simulink model "nanogrid_model"  (R2022a)
settings: Solver=VariableStepAuto  StartTime=0.0  StopTime=86000  RelTol=1e-3
undefined symbols (not defined in the file): Ion, Lithium, sigbuilder_block
libraries: spsCurrentMeasurementLib x18, spsControlledCurrentSourceLib x16, spsVoltageMeasurementLib x12, spsParallelRLCBranchLib x2, spsVariableResistorLib x2, spsBatteryLib x2, spsPVArrayLib x2, spsControlledVoltageSourceLib x1, spsSeriesRLCBranchLib x1, spspowerguiLib x1
(part 1 of 2)
settings Model: SnapshotBufferSize=10000  PacingRate=10  Creator=mhenk  LastModifiedBy=mhenk

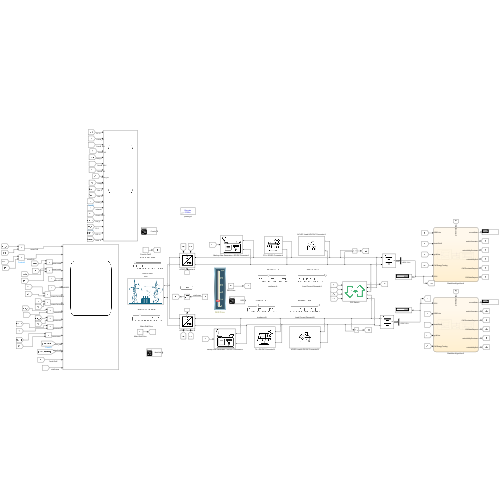
[thumbnail: Simulink's stored preview of the top-level diagram]
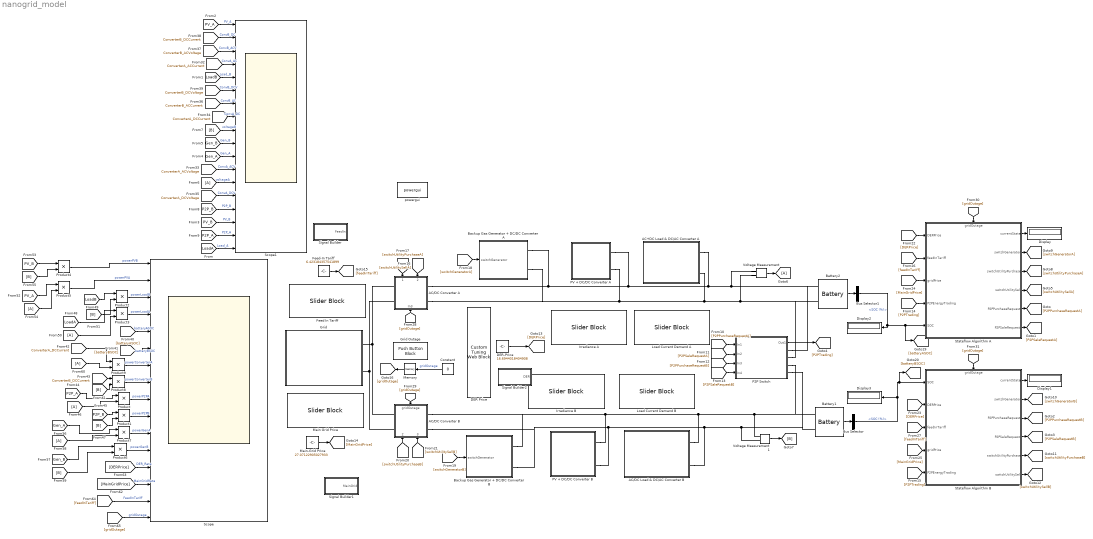
== system nanogrid_model ==
  AC+DC Load & DC/AC Converter A : Subsystem
      mask Display: image('C:\Users\mhenk\Desktop\Data Sync\Documents\education\HSU-UniBwH\Master Thesis\MatLab\own stuff\matlab icons\house load icon.png'); % Use "Edit Image" on toolstrip to change.
  AC/DC Converter A : Subsystem
      settings: PortSchema="{\"entries\":[{\"content\":{\"sides\":[{\"content\":{\"connectorIds\":[\"LConn1\",\"LConn2\"]},\"type\":\"ConnectorPlacement.EquallySpacedRectSide\",\"uuid\":\"d108abb1-5086-446c-b15f-f019b5d6e838\"},{\"content\":{\"connectorIds\":[\"RConn1\",\"RConn2\"],\"side\":\"RIGHT\"},\"type\":\"ConnectorPlacement.EquallySpacedRectSide\",\"uuid\":\"21957a4b-95ce-4ceb-ba72-e824460ef8fd\"},{\"content\":{\"connectorIds\":[\"In1\",\"In2\"],\"side\":\"TOP\"},\"type\":\"ConnectorPlacement.EquallySpacedRectSide\",\"uuid\":\"459c1e26-38cf-4009-a7ae-852720303eb2\"},{\"content\":{\"connectorIds\":[\"In3\"],\"side\":\"BOTTOM\"},\"type\":\"ConnectorPlacement.EquallySpacedRectSide\",\"uuid\":\"e1e3ddba-a993-4c48-8674-2bf20986e444\"}]},\"type\":\"ConnectorPlacement.EquallySpacedConnector\",\"uuid\":\"dcdecdb1-f7ff-4942-94d1-dadc92311a87\"}],\"packageUris\":[\"http://schema.mathworks.com/mf0/Connector/R2020b\"],\"version\":\"1.0\"}"
      mask Display: image('C:\Users\mhenk\Desktop\Data Sync\Documents\education\HSU-UniBwH\Master Thesis\MatLab\own stuff\matlab icons\ac dc converter.png'); % Use "Edit Image" on toolstrip to change.
  AC/DC Converter B : Subsystem
      settings: PortSchema="{\"entries\":[{\"content\":{\"sides\":[{\"content\":{\"connectorIds\":[\"LConn1\",\"LConn2\"]},\"type\":\"ConnectorPlacement.EquallySpacedRectSide\",\"uuid\":\"d108abb1-5086-446c-b15f-f019b5d6e838\"},{\"content\":{\"connectorIds\":[\"RConn1\",\"RConn2\"],\"side\":\"RIGHT\"},\"type\":\"ConnectorPlacement.EquallySpacedRectSide\",\"uuid\":\"21957a4b-95ce-4ceb-ba72-e824460ef8fd\"},{\"content\":{\"connectorIds\":[\"In1\"],\"side\":\"TOP\"},\"type\":\"ConnectorPlacement.EquallySpacedRectSide\",\"uuid\":\"459c1e26-38cf-4009-a7ae-852720303eb2\"},{\"content\":{\"connectorIds\":[\"In2\",\"In3\"],\"side\":\"BOTTOM\"},\"type\":\"ConnectorPlacement.EquallySpacedRectSide\",\"uuid\":\"e1e3ddba-a993-4c48-8674-2bf20986e444\"}]},\"type\":\"ConnectorPlacement.EquallySpacedConnector\",\"uuid\":\"dcdecdb1-f7ff-4942-94d1-dadc92311a87\"}],\"packageUris\":[\"http://schema.mathworks.com/mf0/Connector/R2020b\"],\"version\":\"1.0\"}"
      mask Display: image('C:\Users\mhenk\Desktop\Data Sync\Documents\education\HSU-UniBwH\Master Thesis\MatLab\own stuff\matlab icons\ac dc converter.png'); % Use "Edit Image" on toolstrip to change.
  AC/DC Load & DC/AC Converter B : Subsystem
      mask Display: image('C:\Users\mhenk\Desktop\Data Sync\Documents\education\HSU-UniBwH\Master Thesis\MatLab\own stuff\matlab icons\house load icon.png'); % Use "Edit Image" on toolstrip to change.
  Backup Gas Generator + DC/DC Converter A : Subsystem
      mask Display: image('C:\Users\mhenk\Desktop\Data Sync\Documents\education\HSU-UniBwH\Master Thesis\MatLab\own stuff\matlab icons\gas generator.jpg'); % Use "Edit Image" on toolstrip to change.
  Backup Gas Generator + DC/DC Converter B : Subsystem
      mask Display: image('C:\Users\mhenk\Desktop\Data Sync\Documents\education\HSU-UniBwH\Master Thesis\MatLab\own stuff\matlab icons\gas generator.jpg'); % Use "Edit Image" on toolstrip to change.
  Battery1 : spsBatteryLib/Battery  BatType=Lithium-Ion  ShowTempParam=off  ThermalPreset="12.8V  40Ah  (LiFeMgPO4)"  ShowAgeParam=off  NomV=24  NomQ=500  SOC=1.1  Batt_Tr=30  PresetModel=on  MaxQ=500  MinV=18  FullV=27.9357  Dis_rate=217.3913  R=0.00048  Normal_OP=452.1739  expZone="[25.9293      24.5652]"  current=[6.5 13 32.5]  Units=Time  Tci=20  NomT=20  T2=0  MaxQ2=36  FullV2=13  Normal_OP2=11.7  expZone2="[12.67            4]"  Rca=0.6411  ti=4880  Dp=0  Neq0=0  Tsim=1e6  Ta1=25  Qeol=5.4*0.9  Reol=0.013333*1.2  Char_age=[2.3478, 3]  Dis_age=[2.3478, 10]  N1=1500  N2=10500  N3=1000  N4=1400  Ta2=45  N5=950
  Battery2 : spsBatteryLib/Battery  BatType=Lithium-Ion  ShowTempParam=off  ThermalPreset="12.8V  40Ah  (LiFeMgPO4)"  ShowAgeParam=off  NomV=24  NomQ=500  SOC=99  Batt_Tr=30  PresetModel=on  MaxQ=500  MinV=18  FullV=27.9357  Dis_rate=217.3913  R=0.00048  Normal_OP=452.1739  expZone="[25.9293      24.5652]"  current=[6.5 13 32.5]  Units=Time  Tci=20  NomT=20  T2=0  MaxQ2=36  FullV2=13  Normal_OP2=11.7  expZone2="[12.67            4]"  Rca=0.6411  ti=4880  Dp=0  Neq0=0  Tsim=1e6  Ta1=25  Qeol=5.4*0.9  Reol=0.013333*1.2  Char_age=[2.3478, 3]  Dis_age=[2.3478, 10]  N1=1500  N2=10500  N3=1000  N4=1400  Ta2=45  N5=950
  Bus Selector : BusSelector  OutputSignals=SOC (%)
  Bus Selector1 : BusSelector  OutputSignals=SOC (%)
  Constant : Constant  Value=0
  DER Price : CustomTuningWebBlock  LabelPosition=Hide  ShowInitialText=on  Configuration="{\"type\":\"LinearGauge\",\"settings\":{\"BindingType\":\"param\",\"aspectRatio\":3.7777777777777777,\"backgroundColor\":[0,0,0,\"1\"],\"backgroundOffset\":0,\"backgroundOpacity\":1,\"fixedAspectRatio\":\"on\",\"foregroundColor\":[252,252,196],\"orientation\":\"vertical\",\"showBackgroundColor\":false,\"value\":0},\"components\":[{\"name\":\"LinearScaleComponent\",\"settings\":{\"bounds\":{\"max\":100,\"min\":1,\"tickInterval\":\"auto\"},\"internalTickHeightScaleFactor\":0.5,\"labelColor\":[255,255,200],\"labelFont\":{\"font\":\"Arial\",\"fontSize\":12},\"labelTransparency\":1,\"needleImage\":{\"size\":[596,842],\"src\":\"data:image/svg+xml;base64,PD94bWwgdmVyc2lvbj0iMS4wIiBlbmNvZGluZz0idXRmLTgiPz4NCjwhLS0gR2VuZXJhdG9yOiBBZG9iZSBJbGx1c3RyYXRvciAyNS4wLjAsIFNWRyBFeHBvcnQgUGx1Zy1JbiAuIFNWRyBWZXJzaW9uOiA2LjAwIEJ1aWxkIDApICAtLT4NCjxzdmcgdmVyc2lvbj0iMS4xIg0KCSBpZD0ic3ZnOCIgeG1sbnM6Y2M9Imh0dHA6Ly9jcmVhdGl2ZWNvbW1vbnMub3JnL25zIyIgeG1sbnM6ZGM9Imh0dHA6Ly9wdXJsLm9yZy9kYy9lbGVtZW50cy8xLjEvIiB4bWxuczppbmtzY2FwZT0iaHR0cDovL3d3dy5pbmtzY2FwZS5vcmcvbmFtZXNw ...(+2420 chars)\",\"srcOrientation\":\"horizontal\"},\"needleOffset\":[0.0642123287671233,-0.8044596912521441],\"needleSize\":{\"height\":0.07668067226890757,\"width\":0.4337797619047619},\"position\":[0.03607382550335571,0.2824519230769231,0.6089743589743589,0.9195679530201343],\"referencePoint\":\"auto\",\"scaleColors\":[],\"scaleColorsSize\":0.2,\"scaleDirection\":\"BT\",\"showLabels\":1,\"showMinorTicks\":0,\"showSpanLine\":1,\"showTicks\":1,\"tickColor\":[252,252,197],\"tickTransparency\":1,\"valueBarColor\":[0,114,189],\"valueBarOffset\":-0.27,\"valueBarSize\":0.1,\"valueBarTransparency\":1}},{\"name\":\"BackgroundImageComponent\",\"settings\":{\"image\":{\"size\":[380,101],\"src\":\"data:image/svg+xml;base64,PHN2ZyB4bWxucz0iaHR0cDovL3d3dy53My5vcmcvMjAwMC9zdmciIHhtbG5zOnhsaW5rPSJodHRwOi8vd3d3LnczLm9yZy8xOTk5L3hsaW5rIiB2aWV3Qm94PSIwIDAgMzgwIDEwMSI+PGRlZnM+PHN0eWxlPi5jbHMtMXtmaWxsOiMwMDJiNDI7fS5jbHMtMntmaWxsOiM0MjcwODI7fS5jbHMtM3tmaWxsOnVybCgjcmFkaWFsLWdyYWRpZW50KTt9LmNscy00e2ZpbGw6I2M4YzhjODtzdHJva2U6IzAwMDt9PC9zdHlsZT48cmFkaWFsR3JhZGllbnQgaWQ9InJhZGlhbC1ncmFkaWVudCIgY3g9IjE5MCIgY3k9IjUwLjUiIHI9IjI2OS4yMSIgZ3JhZGllbnRVbml0cz0idXNlclNwYWNlT25Vc2UiPjxzdG9wIG9mZnNldD0iMC4wMSIgc3RvcC1jb2xvcj0iIzNlNGY1OCIvPjxzdG9wIG9mZnNldD0iMC4wNiIgc3RvcC1jb2xvcj0iIzQ0NTc2MSIvPjxzdG9wIG9mZnNldD0iMC4xNSIgc3RvcC1jb2xvcj0iIzU1NmE3NiIvPjxzdG9wIG9mZnNldD0iMC4yNSIgc3RvcC1jb2xvcj0iIzZkODg5NSIvPjxzdG9wIG9mZnNldD0iMC4zOCIgc3RvcC1jb2xvcj0iIzhmYjJjMyIvPjxzdG9wIG9mZnNldD0iMC41MiIgc3RvcC1jb2xvcj0iI2I2ZTRmYSIvPjxzdG9wIG9mZnNldD0iMSIgc3RvcC1jb2xvcj0iIzE1NDY1NyIvPjwvcmFkaWFsR3JhZGllbnQ+PC9kZWZzPjxnIGlkPSJmcmFtZSI+PGcgaWQ9IkxheWVyXzIiIGRhdGEtbmFtZT0iTGF5ZXIgMiI+PGcgaWQ9IkxheWVyXzEtMiIgZGF0YS1uYW1lPSJMYXllciAxLTIiPjxyZWN0IGlkPSJyZWN0MTAzNiIgY2xhc3M9ImNscy0xIiB4PSIxMSIgeT0iMTEiIHdpZHRoPSIzNTgiIGhlaWdodD0iNzkiLz48cGF0aCBpZD0icGF0aDEwMzgiIGNsYXNzPSJjbHMtMiIgZD0iTTgsOFY5M0gzNzJWOFpNMzY5LDkwSDExVjExSDM2OVoiLz48cGF0aCBpZD0icGF0aDEwNDAiIGNsYXNzPSJjbHMtMyIgZD0iTTAsMFYxMDFIMzgwVjBaTTM3Miw5M0g4VjhIMzcyWiIvPjwvZz48L2c+PC9nPjxnIGlkPSJ0cmFjayI+PHBhdGggaWQ9InJlY3QxNjExIiBjbGFzcz0iY2xzLTQiIGQ9Ik0zMy4zNywyNi41OUgzNDYuNjNjNCwwLDcuMjUsMi42LDcuMjUsNS44MWgwYzAsMy4yMS0zLjI1LDUuODItNy4yNSw1LjgySDMzLjM3Yy00LDAtNy4yNS0yLjYxLTcuMjUtNS44MmgwQzI2LjEyLDI5LjE5LDI5LjM3LDI2LjU5LDMzLjM3LDI2LjU5WiIvPjwvZz48L3N2Zz4=\",\"srcOrientation\":\"horizontal\"},\"position\":[0,0,1,1],\"scaleMode\":\"0\"}},{\"name\":\"ForegroundImageComponent\",\"settings\":{\"image\":{\"size\":[0,0],\"src\":\"default\",\"srcOrientation\":[]},\"isForeground\":1,\"position\":[0,0,1,1],\"scaleMode\":\"0\"}}]}"
  DER-Price : Constant  Value=16.6944018404908
  Display{,1..3} (4 alike) : Display
  Feed In Tariff : SliderBlock  ScaleMin=1
  Feed-In Tariff : Constant  Value=6.423184357541899
  From{6,46,50,54,58,60} (6 alike) : From
  Goto6 : Goto
  Grid : Subsystem
      mask Display: image('C:\Users\mhenk\Desktop\Data Sync\Documents\education\HSU-UniBwH\Master Thesis\MatLab\own stuff\matlab icons\power grid transformer substation.jpg'); % Use "Edit Image" on toolstrip to change.
  Grid Outage : PushButtonBlock  ButtonType=Latch  OffValue=0.000000
  Irradiance A : SliderBlock  ScaleMax=1000
  Irradiance B : SliderBlock  ScaleMax=1000
  Load Current Demand A : SliderBlock
  Load Current Demand B : SliderBlock
  Main Grid Price : SliderBlock  ScaleMin=1
  Main-Grid Price : Constant  Value=27.07122905027933
  Memory : Memory
  P2P Switch : Subsystem
      mask Display: image('C:\Users\mhenk\Desktop\Data Sync\Documents\education\HSU-UniBwH\Master Thesis\MatLab\own stuff\matlab icons\p2p.png'); % Use "Edit Image" on toolstrip to change.
  PV + DC/DC Converter A : Subsystem
      mask Display: image('C:\Users\mhenk\Desktop\Data Sync\Documents\education\HSU-UniBwH\Master Thesis\MatLab\own stuff\matlab icons\pv icon.png'); % Use "Edit Image" on toolstrip to change.
  PV + DC/DC Converter B : Subsystem
      mask Display: image('C:\Users\mhenk\Desktop\Data Sync\Documents\education\HSU-UniBwH\Master Thesis\MatLab\own stuff\matlab icons\pv icon.png'); % Use "Edit Image" on toolstrip to change.
  Product{,1..9} (10 alike) : Product
  Scope : Scope  NumInputPorts=16
  Scope1 : Scope  NumInputPorts=18
  Signal Builder : Subsystem  Tag=STV Subsys  LoadFcn=sigbuilder_block('load');  StartFcn=sigbuilder_block('start');  StopFcn=sigbuilder_block('stop');  ClipboardFcn=sigbuilder_block('clipboard');  mask(Sigbuilder block){tuvar=[0:10]}
      mask help: Simulink:masks:SigbuilderBlock_MD
      mask init:
      | if ~strcmp(get_param(bdroot(gcbh),'SimulationStatus'),'stopped') tuvar = sigbuilder_block('maskInit'); end
      settings: CopyFcn=sigbuilder_block('copy');  DeleteFcn=sigbuilder_block('delete');  ModelCloseFcn=sigbuilder_block('modelClose');  PreSaveFcn=sigbuilder_block('preSave');  PauseFcn=sigbuilder_block('pause');  ContinueFcn=sigbuilder_block('continue');  NameChangeFcn=sigbuilder_block('namechange');  OpenFcn=sigbuilder_block('open',[426.6 153 550.8 400.2 ]);  CloseFcn=sigbuilder_block('close');
      mask Display: plot(0, 0, 100, 100,[2, 2, 32, 32, 2], [68, 8, 8, 68, 68],[32, 2], [38, 38], [32, 19, 2],[53, 60, 44], [32, 17, 17, 2],[16, 16, 31, 31]);txt = getActiveGroup(gcbh);text(2, 100, txt,'verticalAlignment', 'top');
  Signal Builder1 : Subsystem  Tag=STV Subsys  LoadFcn=sigbuilder_block('load');  StartFcn=sigbuilder_block('start');  StopFcn=sigbuilder_block('stop');  ClipboardFcn=sigbuilder_block('clipboard');  mask(Sigbuilder block){tuvar=[0:10]}
      mask help: Simulink:masks:SigbuilderBlock_MD
      mask init:
      | if ~strcmp(get_param(bdroot(gcbh),'SimulationStatus'),'stopped') tuvar = sigbuilder_block('maskInit'); end
      settings: CopyFcn=sigbuilder_block('copy');  DeleteFcn=sigbuilder_block('delete');  ModelCloseFcn=sigbuilder_block('modelClose');  PreSaveFcn=sigbuilder_block('preSave');  PauseFcn=sigbuilder_block('pause');  ContinueFcn=sigbuilder_block('continue');  NameChangeFcn=sigbuilder_block('namechange');  OpenFcn=sigbuilder_block('open',[426.6 153 550.8 400.2 ]);  CloseFcn=sigbuilder_block('close');
      mask Display: plot(0, 0, 100, 100,[2, 2, 32, 32, 2], [68, 8, 8, 68, 68],[32, 2], [38, 38], [32, 19, 2],[53, 60, 44], [32, 17, 17, 2],[16, 16, 31, 31]);txt = getActiveGroup(gcbh);text(2, 100, txt,'verticalAlignment', 'top');
  Signal Builder2 : Subsystem  Tag=STV Subsys  LoadFcn=sigbuilder_block('load');  StartFcn=sigbuilder_block('start');  StopFcn=sigbuilder_block('stop');  ClipboardFcn=sigbuilder_block('clipboard');  mask(Sigbuilder block){tuvar=[0:10]}
      mask help: Simulink:masks:SigbuilderBlock_MD
      mask init:
      | if ~strcmp(get_param(bdroot(gcbh),'SimulationStatus'),'stopped') tuvar = sigbuilder_block('maskInit'); end
      settings: CopyFcn=sigbuilder_block('copy');  DeleteFcn=sigbuilder_block('delete');  ModelCloseFcn=sigbuilder_block('modelClose');  PreSaveFcn=sigbuilder_block('preSave');  PauseFcn=sigbuilder_block('pause');  ContinueFcn=sigbuilder_block('continue');  NameChangeFcn=sigbuilder_block('namechange');  OpenFcn=sigbuilder_block('open',[426.6 153 550.8 400.2 ]);  CloseFcn=sigbuilder_block('close');
      mask Display: plot(0, 0, 100, 100,[2, 2, 32, 32, 2], [68, 8, 8, 68, 68],[32, 2], [38, 38], [32, 19, 2],[53, 60, 44], [32, 17, 17, 2],[16, 16, 31, 31]);txt = getActiveGroup(gcbh);text(2, 100, txt,'verticalAlignment', 'top');
  Stateflow Algorithm A : Stateflow chart  TreatAsAtomicUnit=on
      settings: PortSchema="{\"entries\":[{\"content\":{\"sides\":[{\"content\":{\"connectorIds\":[\"In3\",\"In4\",\"In5\",\"In6\",\"In2\"]},\"type\":\"ConnectorPlacement.EquallySpacedRectSide\",\"uuid\":\"fa40be95-7d12-4090-b6c9-44da1494b39c\"},{\"content\":{\"connectorIds\":[\"Out1\",\"Out2\",\"Out3\",\"Out4\",\"Out5\",\"Out6\"],\"side\":\"RIGHT\"},\"type\":\"ConnectorPlacement.EquallySpacedRectSide\",\"uuid\":\"baf17cd9-68a7-482b-a40a-ea138c452546\"},{\"content\":{\"connectorIds\":[\"In1\"],\"side\":\"TOP\"},\"type\":\"ConnectorPlacement.EquallySpacedRectSide\",\"uuid\":\"87fda98d-0e45-402d-8086-d8aba4cb4e5b\"}]},\"type\":\"ConnectorPlacement.EquallySpacedConnector\",\"uuid\":\"afd8760f-ef20-4593-b581-61316121c6e0\"}],\"packageUris\":[\"http://schema.mathworks.com/mf0/Connector/R2020b\"],\"version\":\"1.0\"}"
  Stateflow Algorithm B : Stateflow chart  TreatAsAtomicUnit=on
      settings: PortSchema="{\"entries\":[{\"content\":{\"sides\":[{\"content\":{\"connectorIds\":[\"In2\",\"In3\",\"In4\",\"In5\",\"In6\"]},\"type\":\"ConnectorPlacement.EquallySpacedRectSide\",\"uuid\":\"222fe6c9-2492-4286-b2fe-ee0502c7d1b1\"},{\"content\":{\"connectorIds\":[\"Out1\",\"Out2\",\"Out3\",\"Out4\",\"Out5\",\"Out6\"],\"side\":\"RIGHT\"},\"type\":\"ConnectorPlacement.EquallySpacedRectSide\",\"uuid\":\"fe6cecda-2536-4b6e-a5a3-681bec7accbb\"},{\"content\":{\"connectorIds\":[\"In1\"],\"side\":\"TOP\"},\"type\":\"ConnectorPlacement.EquallySpacedRectSide\",\"uuid\":\"dd9ad14a-77c7-4598-a0b7-e283792e3e97\"}]},\"type\":\"ConnectorPlacement.EquallySpacedConnector\",\"uuid\":\"4279e8cf-6645-4663-97ae-cc11306bf231\"}],\"packageUris\":[\"http://schema.mathworks.com/mf0/Connector/R2020b\"],\"version\":\"1.0\"}"
  Voltage Measurement : spsVoltageMeasurementLib/Voltage Measurement  PhasorSimulation=off  OutputType=Complex  PSBequivalent=0
  Voltage Measurement1 : spsVoltageMeasurementLib/Voltage Measurement  PhasorSimulation=off  OutputType=Complex  PSBequivalent=0
  powergui : spspowerguiLib/powergui  Priority=1  SimulationMode=Discrete  SampleTime=0.009  frequency=50  Iterations=50  frequencyindice=0  Pbase=100e6  ErrMax=1e-4  UnitsV=kV  UnitsW=MW  buscounter=0  FunctionMessages=off  echomessages=off  EnableUseOfTLC=off  CurrentSourceSwitches=off  DisableSnubberDevices=off  DisableRonSwitches=off  DisableVfSwitches=off  DisplayEquations=off  AutomaticDiscreteSolvers=off  SolverType=Tustin/Backward Euler (TBE)  Interpol=off  ExternalGateDelay=off  methode=off  Ts=100  x0status=blocks  SPID=on  SwTol=0  HookPort=off  NonlinearTolerance=1e-4  nMaxIteration=100  ContinueOnMaxIteration=off  RestoreLinks=warning  ResistiveCurrentMeasurement=off  Frange=[0:2:500]  Ylog=off  Xlog=on  ShowGrid=off  save=off  variable=ZData  structure=0  ZoomFFT=off  StartTime=0.0  cycles=1  DisplayStyle=1  fundamental=60  FreqAxis=off  MaxFrequency=1000  frequencyindicesteady=1  RmsSteady=1  display=off
  wires:
  Battery1/1 -> Bus Selector/1
  Battery2/1 -> Bus Selector1/1
  Bus Selector/1 -> [batteryBSOC], Stateflow Algorithm B/2(SOC), Display3/1  "<SOC (%)>"
  Bus Selector1/1 -> [batteryASOC], Stateflow Algorithm A/2(SOC), Display2/1  "<SOC (%)>"
  Voltage Measurement/1 -> Goto6/1
  Stateflow Algorithm A/1(currentState) -> Display/1
  Stateflow Algorithm B/1(currentState) -> Display1/1
  Voltage Measurement1/1 -> [B]
  Stateflow Algorithm A/5(P2PPurchaseRequest) -> [P2PPurchaseRequestA]
  [P2PPurchaseRequestA] -> P2P Switch/1(In1)
  [P2PSaleRequestA] -> P2P Switch/2(In2)
  Stateflow Algorithm A/6(P2PSaleRequest) -> [P2PSaleRequestA]
  Stateflow Algorithm B/3(P2PPurchaseRequest) -> [P2PPurchaseRequestB]
  [P2PPurchaseRequestB] -> P2P Switch/3(In3)
  Stateflow Algorithm B/4(P2PSaleRequest) -> [P2PSaleRequestB]
  [P2PSaleRequestB] -> P2P Switch/4(In4)
  [P2PTrading] -> Stateflow Algorithm A/6(P2PEnergyTrading)
  [P2PTrading] -> Stateflow Algorithm B/6(P2PEnergyTrading)
  P2P Switch/1(Out1) -> [P2PTrading]
  Stateflow Algorithm A/4(switchUtilitySell) -> [switchUtilitySellA]
  [switchUtilitySellA] -> AC/DC Converter A/2(switchGridSell)
  [switchUtilityPurchaseA] -> AC/DC Converter A/1(switchGridPurchase)
  Stateflow Algorithm A/3(switchUtilityPurchase) -> [switchUtilityPurchaseA]
  Stateflow Algorithm A/2(switchGenerator) -> [switchGeneratorA]
  [switchGeneratorA] -> Backup Gas Generator + DC/DC Converter A/1(switchGenerator)
  [switchGeneratorB] -> Backup Gas Generator + DC/DC Converter B/1(switchGenerator)
  Stateflow Algorithm B/2(switchGenerator) -> [switchGeneratorB]
  Stateflow Algorithm B/5(switchUtilityPurchase) -> [switchUtilityPurchaseB]
  [switchUtilityPurchaseB] -> AC/DC Converter B/2(switchGridPurchase)
  [switchUtilitySellB] -> AC/DC Converter B/3(switchGridSell)
  Stateflow Algorithm B/6(switchUtilitySell) -> [switchUtilitySellB]
  [DERPrice] -> Stateflow Algorithm A/3(DERPrice)
  [DERPrice] -> Stateflow Algorithm B/3(DERPrice)
  [MainGridPrice] -> Stateflow Algorithm A/5(gridPrice)
  [MainGridPrice] -> Stateflow Algorithm B/5(gridPrice)
  [feedInTariff] -> Stateflow Algorithm A/4(feedInTariff)
  [feedInTariff] -> Stateflow Algorithm B/4(feedInTariff)
  Memory/1 -> [gridOutage]
  [gridOutage] -> AC/DC Converter A/3(In3)
  [gridOutage] -> AC/DC Converter B/1(gridOutage)
  [PV_A] -> Scope1/1  "PV_A"
  [LoadA] -> Scope1/18  "Load_A"
  [LoadB] -> Scope1/5  "Load_B"
  [gridOutage] -> Stateflow Algorithm A/1(gridOutage)
  [gridOutage] -> Stateflow Algorithm B/1(gridOutage)
  [B] -> Product1/2
  [P2P_B] -> Product1/1
  Product1/1 -> Scope/10  "powerP2PB"
  From50/1 -> Product3/2
  [LoadA] -> Product3/1
  [LoadB] -> Product2/1
  [B] -> Product2/2
  [B] -> Product4/2
  [PV_B] -> Product4/1
  From58/1 -> Product7/2
  [Gen_A] -> Product7/1
  [B] -> Product6/2
  [Gen_B] -> Product6/1
  Product7/1 -> Scope/11  "powerGenA"
  Product6/1 -> Scope/12  "powerGenB"
  Product2/1 -> Scope/3  "powerLoadB"
  Product3/1 -> Scope/4  "powerLoadA"
  Product4/1 -> Scope/1  "powerPVB"
  Constant/1 -> Memory/1  "gridOutage"
  [B] -> Product8/2
  [ConverterA_DCCurrent] -> Product9/1
  From60/1 -> Product9/2
  [ConverterB_DCCurrent] -> Product8/1
  Product9/1 -> Scope/7  "powerConverterA"
  Product8/1 -> Scope/8  "powerConverterB"
  [PV_B] -> Scope1/16  "PV_B"
  [Gen_B] -> Scope1/10  "Gen_B"
  [Gen_A] -> Scope1/11  "Gen_A"
  [P2P_B] -> Scope1/15  "P2P_B"
  [P2P_A] -> Scope1/17  "P2P_A"
  From6/1 -> Scope1/13  "voltageA"
  [ConverterA_ACVoltage] -> Scope1/12  "ConvA_ACV"
  [ConverterA_DCCurrent] -> Scope1/8  "ConvA_DC"
  [B] -> Scope1/9  "voltageB"
  [batteryASOC] -> Scope/5  "batteryASOC"
  [ConverterA_DCVoltage] -> Scope1/14  "ConvA_DCV"
  [ConverterA_ACCurrent] -> Scope1/4  "ConvA_AC"
  [ConverterB_ACCurrent] -> Scope1/7  "ConvB_AC"
  [ConverterB_DCCurrent] -> Scope1/2  "ConvB_DC"
  [ConverterB_DCVoltage] -> Scope1/6  "ConvB_DCV"
  [ConverterB_ACVoltage] -> Scope1/3  "ConvB_ACV"
  [P2P_A] -> Product/1
  From46/1 -> Product/2
  Product/1 -> Scope/9  "powerP2PA"
  [PV_A] -> Product5/1
  From54/1 -> Product5/2
  Product5/1 -> Scope/2  "powerPVA"
  [batteryBSOC] -> Scope/6  "batteryBSOC"
  [DERPrice] -> Scope/13  "DER_Rate"
  [MainGridPrice] -> Scope/14  "MainGridRate"
  [feedInTariff] -> Scope/15  "FeedInTariff"
  [gridOutage] -> Scope/16  "gridOutage"
  Feed-In Tariff/1 -> [feedInTariff]
  Main-Grid Price/1 -> [MainGridPrice]
  DER-Price/1 -> [DERPrice]
  connections:
  AC/DC Converter A/RConn1 -- Backup Gas Generator + DC/DC Converter A/RConn1 -- PV + DC/DC Converter A/RConn1 -- AC+DC Load & DC/AC Converter A/LConn1 -- P2P Switch/RConn1 -- Battery2/LConn1 -- Voltage Measurement/LConn1
  AC/DC Converter B/LConn2 -- AC/DC Converter A/LConn2 -- Grid/LConn2
  AC/DC Converter B/LConn1 -- AC/DC Converter A/LConn1 -- Grid/LConn1
  Voltage Measurement1/LConn1 -- Battery1/LConn1 -- P2P Switch/RConn3 -- Backup Gas Generator + DC/DC Converter B/RConn1 -- AC/DC Converter B/RConn1 -- PV + DC/DC Converter B/RConn1 -- AC/DC Load & DC/AC Converter B/RConn1
  Voltage Measurement/LConn2 -- P2P Switch/RConn2 -- Battery2/LConn2 -- AC/DC Converter A/RConn2 -- Backup Gas Generator + DC/DC Converter A/RConn2 -- PV + DC/DC Converter A/RConn2 -- AC+DC Load & DC/AC Converter A/LConn2
  AC/DC Load & DC/AC Converter B/RConn2 -- Battery1/LConn2 -- P2P Switch/RConn4 -- Voltage Measurement1/LConn2 -- Backup Gas Generator + DC/DC Converter B/RConn2 -- AC/DC Converter B/RConn2 -- PV + DC/DC Converter B/RConn2

== system nanogrid_model/AC+DC Load & DC//AC Converter A ==
  AC+DC Load & DC/AC Converter1 : Subsystem
  Current Measurement2 : spsCurrentMeasurementLib/Current Measurement  PhasorSimulation=off  OutputType=Complex  PSBequivalent=0
  Display : Display
  +1 : PMIOPort  Side=Left
  -1 : PMIOPort  Port=2  Side=Left
  tag scope: LoadA=global
  wires:
  Current Measurement2/1 -> Display/1, [LoadA]  "Load A current"
  connections:
  Current Measurement2/LConn1 -- AC+DC Load & DC/AC Converter1/LConn1
  Current Measurement2/RConn1 -- +1/RConn1
  AC+DC Load & DC/AC Converter1/LConn2 -- -1/RConn1

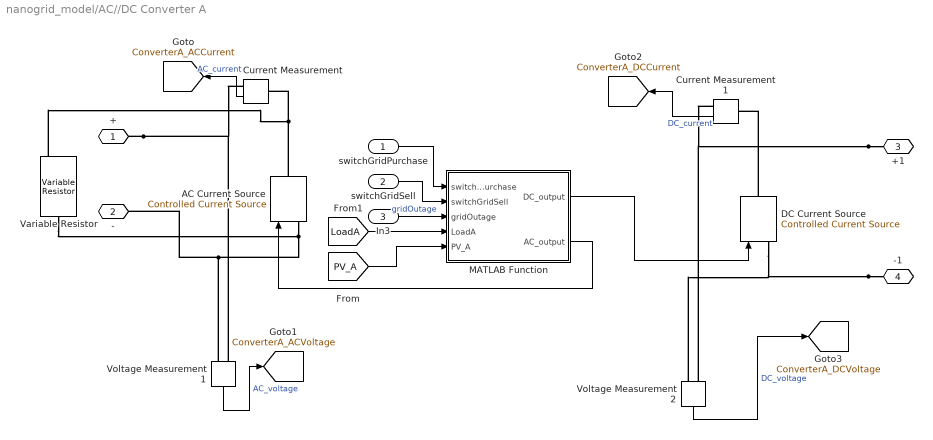
== system nanogrid_model/AC//DC Converter A ==
  switchGridPurchase : Inport
  switchGridSell : Inport  Port=2
  In3 : Inport  Port=3
  AC Current Source : spsControlledCurrentSourceLib/Controlled Current Source  Initialize=on  Source_Type=AC  Amplitude=0  Phase=0  Frequency=60  Measurements=None
  Current Measurement : spsCurrentMeasurementLib/Current Measurement  PhasorSimulation=off  OutputType=Complex  PSBequivalent=0
  Current Measurement1 : spsCurrentMeasurementLib/Current Measurement  PhasorSimulation=off  OutputType=Complex  PSBequivalent=0
  DC Current Source : spsControlledCurrentSourceLib/Controlled Current Source  Initialize=on  Source_Type=DC  Amplitude=0  Phase=0  Frequency=0  Measurements=None
  MATLAB Function : MATLAB Function  TreatAsAtomicUnit=on
  Variable Resistor : spsVariableResistorLib/Variable Resistor  Rabsmin=50e9
      settings: SourceProductBaseCode=PS
  Voltage Measurement1 : spsVoltageMeasurementLib/Voltage Measurement  PhasorSimulation=off  OutputType=Complex  PSBequivalent=0
  Voltage Measurement2 : spsVoltageMeasurementLib/Voltage Measurement  PhasorSimulation=off  OutputType=Complex  PSBequivalent=0
  + : PMIOPort  Side=Left
  - : PMIOPort  Port=2  Side=Left
  +1 : PMIOPort  Port=3  Side=Right
  -1 : PMIOPort  Port=4  Side=Right
  tag scope: ConverterA_ACCurrent=global, ConverterA_ACVoltage=global, ConverterA_DCCurrent=global, ConverterA_DCVoltage=global
  wires:
  MATLAB Function/1(DC_output) -> DC Current Source/1
  Current Measurement/1 -> [ConverterA_ACCurrent]  "AC_current"
  Voltage Measurement1/1 -> [ConverterA_ACVoltage]  "AC_voltage"
  Current Measurement1/1 -> [ConverterA_DCCurrent]  "DC_current"
  Voltage Measurement2/1 -> [ConverterA_DCVoltage]  "DC_voltage"
  MATLAB Function/2(AC_output) -> AC Current Source/1
  switchGridPurchase/1 -> MATLAB Function/1(switchGridPurchase)
  switchGridSell/1 -> MATLAB Function/2(switchGridSell)
  In3/1 -> MATLAB Function/3(gridOutage)  "gridOutage"
  [PV_A] -> MATLAB Function/5(PV_A)
  [LoadA] -> MATLAB Function/4(LoadA)
  connections:
  +/RConn1 -- Current Measurement/RConn1 -- Voltage Measurement1/LConn1
  AC Current Source/LConn1 -- Variable Resistor/RConn1 -- Voltage Measurement1/LConn2 -- -/RConn1
  AC Current Source/RConn1 -- Variable Resistor/LConn1 -- Current Measurement/LConn1
  -1/RConn1 -- Voltage Measurement2/LConn2 -- DC Current Source/LConn1
  +1/RConn1 -- Current Measurement1/RConn1 -- Voltage Measurement2/LConn1
  DC Current Source/RConn1 -- Current Measurement1/LConn1

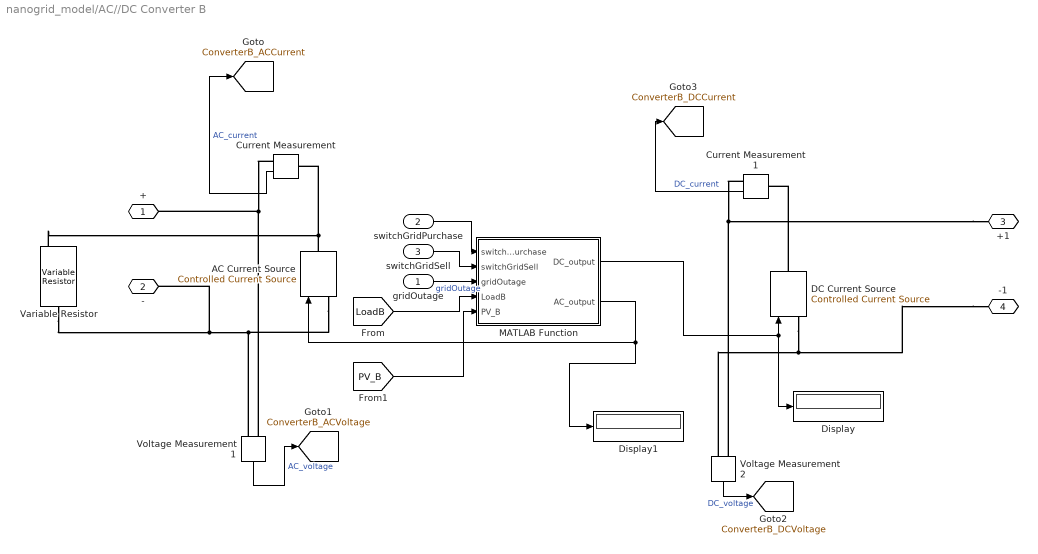
== system nanogrid_model/AC//DC Converter B ==
  gridOutage : Inport
  switchGridPurchase : Inport  Port=2
  switchGridSell : Inport  Port=3
  AC Current Source : spsControlledCurrentSourceLib/Controlled Current Source  Initialize=on  Source_Type=AC  Amplitude=0  Phase=0  Frequency=0  Measurements=None
  Current Measurement : spsCurrentMeasurementLib/Current Measurement  PhasorSimulation=off  OutputType=Complex  PSBequivalent=0
  Current Measurement1 : spsCurrentMeasurementLib/Current Measurement  PhasorSimulation=off  OutputType=Complex  PSBequivalent=0
  DC Current Source : spsControlledCurrentSourceLib/Controlled Current Source  Initialize=on  Source_Type=DC  Amplitude=0  Phase=0  Frequency=0  Measurements=None
  Display : Display
  Display1 : Display
  MATLAB Function : MATLAB Function  TreatAsAtomicUnit=on
  Variable Resistor : spsVariableResistorLib/Variable Resistor  Rabsmin=50e9
      settings: SourceProductBaseCode=PS
  Voltage Measurement1 : spsVoltageMeasurementLib/Voltage Measurement  PhasorSimulation=off  OutputType=Complex  PSBequivalent=0
  Voltage Measurement2 : spsVoltageMeasurementLib/Voltage Measurement  PhasorSimulation=off  OutputType=Complex  PSBequivalent=0
  + : PMIOPort  Side=Left
  - : PMIOPort  Port=2  Side=Left
  +1 : PMIOPort  Port=3  Side=Right
  -1 : PMIOPort  Port=4  Side=Right
  tag scope: ConverterB_ACCurrent=global, ConverterB_ACVoltage=global, ConverterB_DCCurrent=global, ConverterB_DCVoltage=global
  wires:
  MATLAB Function/1(DC_output) -> Display/1, DC Current Source/1
  Current Measurement/1 -> [ConverterB_ACCurrent]  "AC_current"
  Voltage Measurement1/1 -> [ConverterB_ACVoltage]  "AC_voltage"
  Current Measurement1/1 -> [ConverterB_DCCurrent]  "DC_current"
  Voltage Measurement2/1 -> [ConverterB_DCVoltage]  "DC_voltage"
  MATLAB Function/2(AC_output) -> Display1/1, AC Current Source/1
  switchGridPurchase/1 -> MATLAB Function/1(switchGridPurchase)
  switchGridSell/1 -> MATLAB Function/2(switchGridSell)
  gridOutage/1 -> MATLAB Function/3(gridOutage)  "gridOutage"
  [LoadB] -> MATLAB Function/4(LoadB)
  [PV_B] -> MATLAB Function/5(PV_B)
  connections:
  +/RConn1 -- Current Measurement/RConn1 -- Voltage Measurement1/LConn1
  AC Current Source/LConn1 -- Variable Resistor/RConn1 -- -/RConn1 -- Voltage Measurement1/LConn2
  AC Current Source/RConn1 -- Current Measurement/LConn1 -- Variable Resistor/LConn1
  -1/RConn1 -- DC Current Source/LConn1 -- Voltage Measurement2/LConn2
  +1/RConn1 -- Current Measurement1/RConn1 -- Voltage Measurement2/LConn1
  DC Current Source/RConn1 -- Current Measurement1/LConn1

== system nanogrid_model/AC//DC Load & DC//AC Converter B ==
  AC/DC Load & DC/AC Converter : Subsystem
  Current Measurement3 : spsCurrentMeasurementLib/Current Measurement  PhasorSimulation=off  OutputType=Complex  PSBequivalent=0
  +1 : PMIOPort  Side=Right
  -1 : PMIOPort  Port=2  Side=Right
  tag scope: LoadB=global
  wires:
  Current Measurement3/1 -> [LoadB]  "Load B Current"
  connections:
  Current Measurement3/LConn1 -- AC/DC Load & DC/AC Converter/LConn1
  Current Measurement3/RConn1 -- +1/RConn1
  AC/DC Load & DC/AC Converter/LConn2 -- -1/RConn1

== system nanogrid_model/Backup Gas Generator + DC//DC Converter A ==
  switchGenerator : Inport
  Backup Gas Generator + DC/DC Converter1 : Subsystem
      settings: PortSchema="{\"entries\":[{\"content\":{\"sides\":[{\"content\":{\"connectorIds\":[]},\"type\":\"ConnectorPlacement.EquallySpacedRectSide\",\"uuid\":\"2b2976e8-5e35-4ebb-b89a-c6bd5733880a\"},{\"content\":{\"connectorIds\":[\"RConn1\",\"RConn2\"],\"side\":\"RIGHT\"},\"type\":\"ConnectorPlacement.EquallySpacedRectSide\",\"uuid\":\"3f5067af-896c-4e1f-b6f7-733e5cdc76c1\"},{\"content\":{\"connectorIds\":[\"In1\"],\"side\":\"TOP\"},\"type\":\"ConnectorPlacement.EquallySpacedRectSide\",\"uuid\":\"f222cd72-c1be-4f44-b61b-d0eaed55e8e5\"},{\"content\":{\"connectorIds\":[],\"side\":\"BOTTOM\"},\"type\":\"ConnectorPlacement.EquallySpacedRectSide\",\"uuid\":\"38c9aab2-4887-46b3-83a5-02a238a37665\"}]},\"type\":\"ConnectorPlacement.EquallySpacedConnector\",\"uuid\":\"8be83150-dffc-4bc0-b134-d817f89340a9\"}],\"packageUris\":[\"http://schema.mathworks.com/mf0/Connector/R2020b\"],\"version\":\"1.0\"}"
  Current Measurement : spsCurrentMeasurementLib/Current Measurement  PhasorSimulation=off  OutputType=Complex  PSBequivalent=0
  +1 : PMIOPort  Side=Right
  -1 : PMIOPort  Port=2  Side=Right
  tag scope: Gen_A=global
  wires:
  Current Measurement/1 -> [Gen_A]
  switchGenerator/1 -> Backup Gas Generator + DC/DC Converter1/1(switchGenerator)
  connections:
  Backup Gas Generator + DC/DC Converter1/RConn1 -- Current Measurement/LConn1
  Current Measurement/RConn1 -- +1/RConn1
  Backup Gas Generator + DC/DC Converter1/RConn2 -- -1/RConn1

== system nanogrid_model/Backup Gas Generator + DC//DC Converter B ==
  switchGenerator : Inport
  Backup Gas Generator + DC/DC Converter : Subsystem
      settings: PortSchema="{\"entries\":[{\"content\":{\"sides\":[{\"content\":{\"connectorIds\":[]},\"type\":\"ConnectorPlacement.EquallySpacedRectSide\",\"uuid\":\"2b2976e8-5e35-4ebb-b89a-c6bd5733880a\"},{\"content\":{\"connectorIds\":[\"RConn1\",\"RConn2\"],\"side\":\"RIGHT\"},\"type\":\"ConnectorPlacement.EquallySpacedRectSide\",\"uuid\":\"3f5067af-896c-4e1f-b6f7-733e5cdc76c1\"},{\"content\":{\"connectorIds\":[],\"side\":\"TOP\"},\"type\":\"ConnectorPlacement.EquallySpacedRectSide\",\"uuid\":\"f222cd72-c1be-4f44-b61b-d0eaed55e8e5\"},{\"content\":{\"connectorIds\":[\"In1\"],\"side\":\"BOTTOM\"},\"type\":\"ConnectorPlacement.EquallySpacedRectSide\",\"uuid\":\"38c9aab2-4887-46b3-83a5-02a238a37665\"}]},\"type\":\"ConnectorPlacement.EquallySpacedConnector\",\"uuid\":\"8be83150-dffc-4bc0-b134-d817f89340a9\"}],\"packageUris\":[\"http://schema.mathworks.com/mf0/Connector/R2020b\"],\"version\":\"1.0\"}"
  Current Measurement5 : spsCurrentMeasurementLib/Current Measurement  PhasorSimulation=off  OutputType=Complex  PSBequivalent=0
  +1 : PMIOPort  Side=Right
  -1 : PMIOPort  Port=2  Side=Right
  tag scope: Gen_B=global
  wires:
  Current Measurement5/1 -> [Gen_B]
  switchGenerator/1 -> Backup Gas Generator + DC/DC Converter/1(switchGenerator)
  connections:
  Current Measurement5/RConn1 -- +1/RConn1
  Backup Gas Generator + DC/DC Converter/RConn1 -- Current Measurement5/LConn1
  Backup Gas Generator + DC/DC Converter/RConn2 -- -1/RConn1

== system nanogrid_model/Grid ==
  Constant : Constant  Value=1000
  Controlled Voltage Source : spsControlledVoltageSourceLib/Controlled Voltage Source  Initialize=on  Source_Type=AC  Amplitude=120  Phase=0  Frequency=60  Measurements=None
  Series RLC Branch : spsSeriesRLCBranchLib/Series RLC Branch  LConnTagsString=__new0  RConnTagsString=__new0  BranchType=R  Resistance=1  Inductance=0.9e-9  SetiL0=off  InitialCurrent=0  Capacitance=1e-6  Setx0=off  InitialVoltage=0  Measurements=None
  + : PMIOPort  Side=Left
  - : PMIOPort  Port=2  Side=Left
  wires:
  Constant/1 -> Controlled Voltage Source/1
  connections:
  Controlled Voltage Source/RConn1 -- Series RLC Branch/RConn1
  -/RConn1 -- Controlled Voltage Source/LConn1
  +/RConn1 -- Series RLC Branch/LConn1

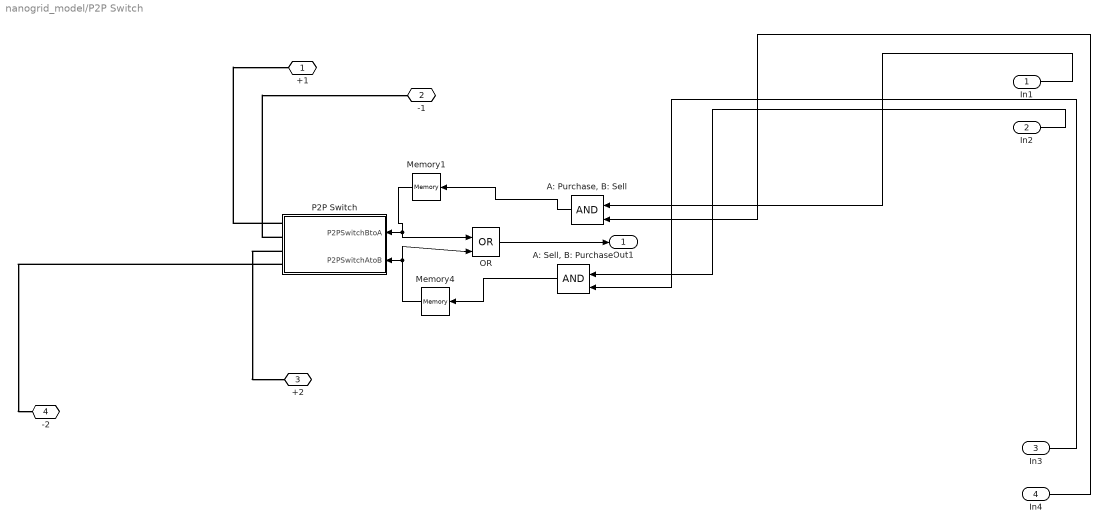
== system nanogrid_model/P2P Switch ==
  In1 : Inport
  In2 : Inport  Port=2
  In3 : Inport  Port=3
  In4 : Inport  Port=4
  "A: Purchase, B: Sell" : Logic  IconShape=distinctive  AllPortsSameDT=off  OutDataTypeStr=boolean
  "A: Sell, B: Purchase" : Logic  IconShape=distinctive  AllPortsSameDT=off  OutDataTypeStr=boolean
  Memory1 : Memory
  Memory4 : Memory
  OR : Logic  Operator=OR  IconShape=distinctive  AllPortsSameDT=off  OutDataTypeStr=boolean
  P2P Switch : Subsystem
  +1 : PMIOPort  Side=Right
  -1 : PMIOPort  Port=2  Side=Right
  +2 : PMIOPort  Port=3  Side=Right
  -2 : PMIOPort  Port=4  Side=Right
  Out1 : Outport
  wires:
  In2/1 -> "A: Sell, B: Purchase"/1
  Memory1/1 -> P2P Switch/1(P2PSwitchBtoA), OR/1
  "A: Sell, B: Purchase"/1 -> Memory4/1
  Memory4/1 -> OR/2, P2P Switch/2(P2PSwitchAtoB)
  "A: Purchase, B: Sell"/1 -> Memory1/1
  In1/1 -> "A: Purchase, B: Sell"/1
  In3/1 -> "A: Sell, B: Purchase"/2
  In4/1 -> "A: Purchase, B: Sell"/2
  OR/1 -> Out1/1
  connections:
  P2P Switch/RConn1 -- +1/RConn1
  P2P Switch/RConn2 -- -1/RConn1
  P2P Switch/RConn3 -- +2/RConn1
  P2P Switch/RConn4 -- -2/RConn1

== system nanogrid_model/PV + DC//DC Converter A ==
  Current Measurement1 : spsCurrentMeasurementLib/Current Measurement  PhasorSimulation=off  OutputType=Complex  PSBequivalent=0
  PV + DC/DC Converter1 : Subsystem
  +1 : PMIOPort  Side=Right
  -1 : PMIOPort  Port=2  Side=Right
  tag scope: PV_A=global
  wires:
  Current Measurement1/1 -> [PV_A]
  connections:
  PV + DC/DC Converter1/RConn1 -- Current Measurement1/LConn1
  Current Measurement1/RConn1 -- +1/RConn1
  PV + DC/DC Converter1/RConn2 -- -1/RConn1

== system nanogrid_model/PV + DC//DC Converter B ==
  Current Measurement4 : spsCurrentMeasurementLib/Current Measurement  PhasorSimulation=off  OutputType=Complex  PSBequivalent=0
  PV + DC/DC Converter : Subsystem
  +1 : PMIOPort  Side=Right
  -1 : PMIOPort  Port=2  Side=Right
  tag scope: PV_B=global
  wires:
  Current Measurement4/1 -> [PV_B]
  connections:
  Current Measurement4/LConn1 -- PV + DC/DC Converter/RConn1
  Current Measurement4/RConn1 -- +1/RConn1
  PV + DC/DC Converter/RConn2 -- -1/RConn1

== system nanogrid_model/Signal Builder ==
  Demux : Demux  Tag=STV Demux  Outputs=1
      settings: DisplayOption=none
  FromWs : FromWorkspace  Tag=STV FromWs  VariableName=tuvar
      SigBuilderData=|
      | common.afterFinalStr = 'Extrapolate'
      | common.sampleTime = 0
      | dataSet.timeRange = [0 82411]
      | dataSet.name = 'Sheet1'
      | sbobj.Groups.Name = 'Sheet1'
      | sbobj.Groups.Signals.Name = 'FeedIn'
      | sbobj.Groups.Signals.XData = [0 3583 7166 10750 14332 17915 21498 25083 28666 32249 35832 39415 42998 46581 50164 53747 57330 60913 65000 68079 71662 75245 78828 82411]
      | sbobj.Groups.Signals.YData = [5 5 5 5 12 12 12 12 12 5 9 9 9 9 7 7 3 3 5 5 5 5 9 9]
  FeedIn : Outport  Tag=STV Outport
  wires:
  Demux/1 -> FeedIn/1
  FromWs/1 -> Demux/1

== system nanogrid_model/Signal Builder1 ==
  Demux : Demux  Tag=STV Demux  Outputs=1
      settings: DisplayOption=none
  FromWs : FromWorkspace  Tag=STV FromWs  VariableName=tuvar
      SigBuilderData=|
      | common.afterFinalStr = 'Extrapolate'
      | common.sampleTime = 0
      | dataSet.timeRange = [0 82411]
      | dataSet.name = 'Sheet1'
      | sbobj.Groups.Name = 'Sheet1'
      | sbobj.Groups.Signals.Name = 'MainGrid'
      | sbobj.Groups.Signals.XData = [0 3583 7166 10750 14332 17915 21498 25083 28666 32249 35832 39415 42998 46581 50164 53747 57330 60913 65000 68079 71662 75245 78828 82411]
      | sbobj.Groups.Signals.YData = [28 32 32 32 28 28 28 28 28 32 32 32 32 28 28 28 28 28 28 32 32 32 32 32]
      | sbobj.Groups.TimeRange = [0 82411]
  MainGrid : Outport  Tag=STV Outport
  wires:
  Demux/1 -> MainGrid/1
  FromWs/1 -> Demux/1

== system nanogrid_model/Signal Builder2 ==
  Demux : Demux  Tag=STV Demux  Outputs=1
      settings: DisplayOption=none
  FromWs : FromWorkspace  Tag=STV FromWs  VariableName=tuvar
      SigBuilderData=|
      | common.afterFinalStr = 'Extrapolate'
      | common.sampleTime = 0
      | dataSet.timeRange = [0 82411]
      | dataSet.name = 'Sheet1'
      | sbobj.Groups.Name = 'Sheet1'
      | sbobj.Groups.Signals.Name = 'DER'
      | sbobj.Groups.Signals.XData = [0 3583 7166 10750 14332 17915 21498 25083 28666 32249 35832 39415 42998 46581 50164 53747 57330 60913 65000 68079 71662 75245 78828 82411]
      | sbobj.Groups.Signals.YData = [20 20 20 20 20 20 20 20 20 20 20 20 20 20 20 20 20 40 40 40 40 40 40 40]
      | sbobj.Groups.TimeRange = [0 82411]
  DER : Outport  Tag=STV Outport
  wires:
  Demux/1 -> DER/1
  FromWs/1 -> Demux/1

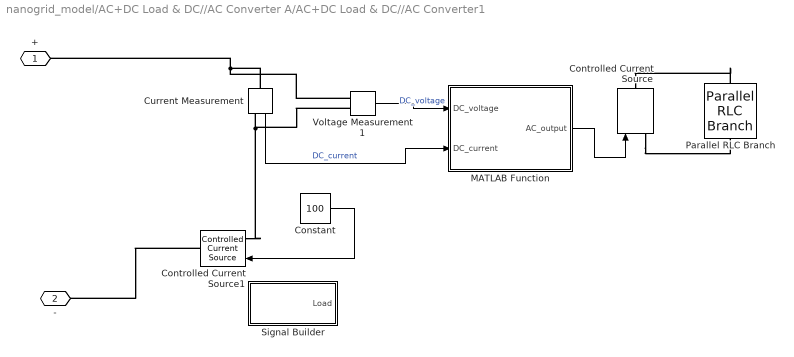
== system nanogrid_model/AC+DC Load & DC//AC Converter A/AC+DC Load & DC//AC Converter1 ==
  Constant : Constant  Value=100
  Controlled Current Source : spsControlledCurrentSourceLib/Controlled Current Source  Initialize=on  Source_Type=AC  Amplitude=0  Phase=0  Frequency=60  Measurements=None
  Controlled Current Source1 : spsControlledCurrentSourceLib/Controlled Current Source  Initialize=on  Source_Type=DC  Amplitude=80  Phase=0  Frequency=60  Measurements=None
  Current Measurement : spsCurrentMeasurementLib/Current Measurement  PhasorSimulation=off  OutputType=Complex  PSBequivalent=0
  MATLAB Function : MATLAB Function  TreatAsAtomicUnit=on
  Parallel RLC Branch : spsParallelRLCBranchLib/Parallel RLC Branch  LConnTagsString=a  RConnTagsString=__new0  BranchType=RL  Resistance=1e3  Inductance=1e-3  SetiL0=off  InitialCurrent=0  Capacitance=1e-6  Setx0=off  InitialVoltage=0  Measurements=None
  Signal Builder : Subsystem  Tag=STV Subsys  LoadFcn=sigbuilder_block('load');  StartFcn=sigbuilder_block('start');  StopFcn=sigbuilder_block('stop');  ClipboardFcn=sigbuilder_block('clipboard');  mask(Sigbuilder block){tuvar=[0:10]}
      mask help: Simulink:masks:SigbuilderBlock_MD
      mask init:
      | if ~strcmp(get_param(bdroot(gcbh),'SimulationStatus'),'stopped') tuvar = sigbuilder_block('maskInit'); end
      settings: CopyFcn=sigbuilder_block('copy');  DeleteFcn=sigbuilder_block('delete');  ModelCloseFcn=sigbuilder_block('modelClose');  PreSaveFcn=sigbuilder_block('preSave');  PauseFcn=sigbuilder_block('pause');  ContinueFcn=sigbuilder_block('continue');  NameChangeFcn=sigbuilder_block('namechange');  OpenFcn=sigbuilder_block('open',[437.6 199.2 550.4 400 ]);  CloseFcn=sigbuilder_block('close');
      mask Display: plot(0, 0, 100, 100,[2, 2, 32, 32, 2], [68, 8, 8, 68, 68],[32, 2], [38, 38], [32, 19, 2],[53, 60, 44], [32, 17, 17, 2],[16, 16, 31, 31]);txt = getActiveGroup(gcbh);text(2, 100, txt,'verticalAlignment', 'top');
  Voltage Measurement1 : spsVoltageMeasurementLib/Voltage Measurement  PhasorSimulation=off  OutputType=Complex  PSBequivalent=0
  + : PMIOPort  Side=Left
  - : PMIOPort  Port=2  Side=Left
  wires:
  Current Measurement/1 -> MATLAB Function/2(DC_current)  "DC_current"
  Voltage Measurement1/1 -> MATLAB Function/1(DC_voltage)  "DC_voltage"
  MATLAB Function/1(AC_output) -> Controlled Current Source/1
  Constant/1 -> Controlled Current Source1/1
  connections:
  Voltage Measurement1/LConn1 -- Current Measurement/LConn1 -- +/RConn1
  Voltage Measurement1/LConn2 -- Controlled Current Source1/LConn1 -- Current Measurement/RConn1
  Parallel RLC Branch/LConn1 -- Controlled Current Source/RConn1
  Controlled Current Source/LConn1 -- Parallel RLC Branch/RConn1
  Controlled Current Source1/RConn1 -- -/RConn1

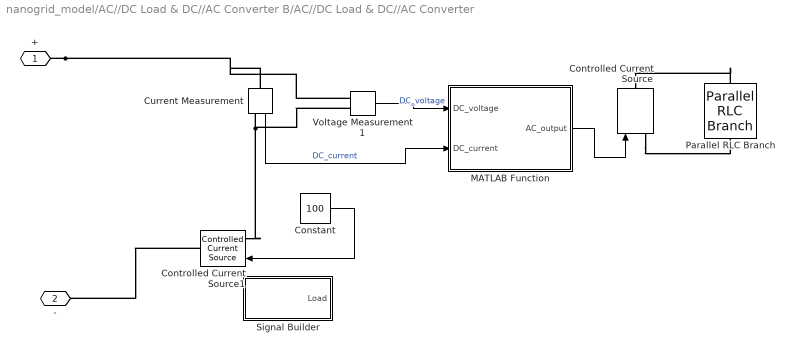
== system nanogrid_model/AC//DC Load & DC//AC Converter B/AC//DC Load & DC//AC Converter ==
  Constant : Constant  Value=100
  Controlled Current Source : spsControlledCurrentSourceLib/Controlled Current Source  Initialize=on  Source_Type=AC  Amplitude=0  Phase=0  Frequency=60  Measurements=None
  Controlled Current Source1 : spsControlledCurrentSourceLib/Controlled Current Source  Initialize=on  Source_Type=DC  Amplitude=80  Phase=0  Frequency=60  Measurements=None
  Current Measurement : spsCurrentMeasurementLib/Current Measurement  PhasorSimulation=off  OutputType=Complex  PSBequivalent=0
  MATLAB Function : MATLAB Function  TreatAsAtomicUnit=on
  Parallel RLC Branch : spsParallelRLCBranchLib/Parallel RLC Branch  LConnTagsString=a  RConnTagsString=__new0  BranchType=RL  Resistance=1e3  Inductance=1e-3  SetiL0=off  InitialCurrent=0  Capacitance=1e-6  Setx0=off  InitialVoltage=0  Measurements=None
  Signal Builder : Subsystem  Tag=STV Subsys  LoadFcn=sigbuilder_block('load');  StartFcn=sigbuilder_block('start');  StopFcn=sigbuilder_block('stop');  ClipboardFcn=sigbuilder_block('clipboard');  mask(Sigbuilder block){tuvar=[0:10]}
      mask help: Simulink:masks:SigbuilderBlock_MD
      mask init:
      | if ~strcmp(get_param(bdroot(gcbh),'SimulationStatus'),'stopped') tuvar = sigbuilder_block('maskInit'); end
      settings: CopyFcn=sigbuilder_block('copy');  DeleteFcn=sigbuilder_block('delete');  ModelCloseFcn=sigbuilder_block('modelClose');  PreSaveFcn=sigbuilder_block('preSave');  PauseFcn=sigbuilder_block('pause');  ContinueFcn=sigbuilder_block('continue');  NameChangeFcn=sigbuilder_block('namechange');  OpenFcn=sigbuilder_block('open',[437.4 84 550.8 400.2 ]);  CloseFcn=sigbuilder_block('close');
      mask Display: plot(0, 0, 100, 100,[2, 2, 32, 32, 2], [68, 8, 8, 68, 68],[32, 2], [38, 38], [32, 19, 2],[53, 60, 44], [32, 17, 17, 2],[16, 16, 31, 31]);txt = getActiveGroup(gcbh);text(2, 100, txt,'verticalAlignment', 'top');
  Voltage Measurement1 : spsVoltageMeasurementLib/Voltage Measurement  PhasorSimulation=off  OutputType=Complex  PSBequivalent=0
  + : PMIOPort  Side=Left
  - : PMIOPort  Port=2  Side=Left
  wires:
  MATLAB Function/1(AC_output) -> Controlled Current Source/1
  Current Measurement/1 -> MATLAB Function/2(DC_current)  "DC_current"
  Voltage Measurement1/1 -> MATLAB Function/1(DC_voltage)  "DC_voltage"
  Constant/1 -> Controlled Current Source1/1
  connections:
  +/RConn1 -- Voltage Measurement1/LConn1 -- Current Measurement/LConn1
  Current Measurement/RConn1 -- Voltage Measurement1/LConn2 -- Controlled Current Source1/LConn1
  Controlled Current Source/LConn1 -- Parallel RLC Branch/RConn1
  Controlled Current Source1/RConn1 -- -/RConn1
  Parallel RLC Branch/LConn1 -- Controlled Current Source/RConn1

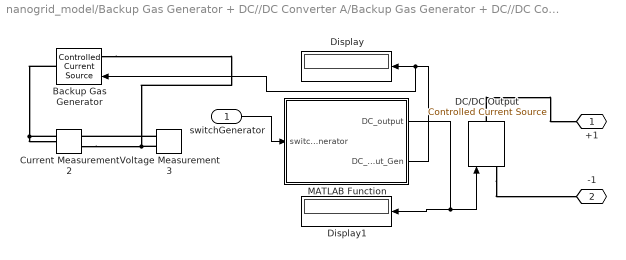
== system nanogrid_model/Backup Gas Generator + DC//DC Converter A/Backup Gas Generator + DC//DC Converter1 ==
  switchGenerator : Inport
  Backup Gas Generator : spsControlledCurrentSourceLib/Controlled Current Source  Initialize=on  Source_Type=DC  Amplitude=100  Phase=0  Frequency=0  Measurements=None
  Current Measurement2 : spsCurrentMeasurementLib/Current Measurement  PhasorSimulation=off  OutputType=Complex  PSBequivalent=0
  DC/DC Output : spsControlledCurrentSourceLib/Controlled Current Source  Initialize=on  Source_Type=DC  Amplitude=0  Phase=0  Frequency=0  Measurements=None
  Display : Display
  Display1 : Display
  MATLAB Function : MATLAB Function  TreatAsAtomicUnit=on
  Voltage Measurement3 : spsVoltageMeasurementLib/Voltage Measurement  PhasorSimulation=off  OutputType=Complex  PSBequivalent=0
  +1 : PMIOPort  Side=Right
  -1 : PMIOPort  Port=2  Side=Right
  wires:
  MATLAB Function/1(DC_output) -> DC/DC Output/1, Display1/1
  switchGenerator/1 -> MATLAB Function/1(switchGenerator)
  MATLAB Function/2(DC_output_Gen) -> Backup Gas Generator/1, Display/1
  connections:
  DC/DC Output/LConn1 -- -1/RConn1
  Voltage Measurement3/LConn1 -- Current Measurement2/LConn1 -- Backup Gas Generator/RConn1
  Voltage Measurement3/LConn2 -- Current Measurement2/RConn1 -- Backup Gas Generator/LConn1
  DC/DC Output/RConn1 -- +1/RConn1

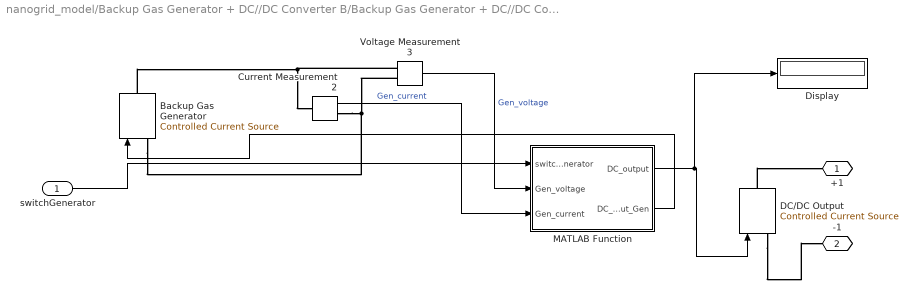
== system nanogrid_model/Backup Gas Generator + DC//DC Converter B/Backup Gas Generator + DC//DC Converter ==
  switchGenerator : Inport
  Backup Gas Generator : spsControlledCurrentSourceLib/Controlled Current Source  Initialize=on  Source_Type=DC  Amplitude=2.3  Phase=0  Frequency=0  Measurements=None
  Current Measurement2 : spsCurrentMeasurementLib/Current Measurement  PhasorSimulation=off  OutputType=Complex  PSBequivalent=0
  DC/DC Output : spsControlledCurrentSourceLib/Controlled Current Source  Initialize=on  Source_Type=DC  Amplitude=0  Phase=0  Frequency=0  Measurements=None
  Display : Display
  MATLAB Function : MATLAB Function  TreatAsAtomicUnit=on
  Voltage Measurement3 : spsVoltageMeasurementLib/Voltage Measurement  PhasorSimulation=off  OutputType=Complex  PSBequivalent=0
  +1 : PMIOPort  Side=Right
  -1 : PMIOPort  Port=2  Side=Right
  wires:
  MATLAB Function/1(DC_output) -> Display/1, DC/DC Output/1
  Voltage Measurement3/1 -> MATLAB Function/2(Gen_voltage)  "Gen_voltage"
  Current Measurement2/1 -> MATLAB Function/3(Gen_current)  "Gen_current"
  switchGenerator/1 -> MATLAB Function/1(switchGenerator)
  MATLAB Function/2(DC_output_Gen) -> Backup Gas Generator/1
  connections:
  DC/DC Output/LConn1 -- -1/RConn1
  Voltage Measurement3/LConn1 -- Backup Gas Generator/RConn1 -- Current Measurement2/LConn1
  Voltage Measurement3/LConn2 -- Backup Gas Generator/LConn1 -- Current Measurement2/RConn1
  DC/DC Output/RConn1 -- +1/RConn1

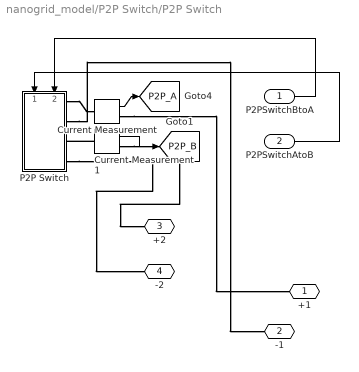
== system nanogrid_model/P2P Switch/P2P Switch ==
  P2PSwitchBtoA : Inport
  P2PSwitchAtoB : Inport  Port=2
  Current Measurement : spsCurrentMeasurementLib/Current Measurement  PhasorSimulation=off  OutputType=Complex  PSBequivalent=0
  Current Measurement1 : spsCurrentMeasurementLib/Current Measurement  PhasorSimulation=off  OutputType=Complex  PSBequivalent=0
  P2P Switch : Subsystem
      settings: PortSchema="{\"entries\":[{\"content\":{\"sides\":[{\"content\":{\"connectorIds\":[]},\"type\":\"ConnectorPlacement.EquallySpacedRectSide\",\"uuid\":\"2b2976e8-5e35-4ebb-b89a-c6bd5733880a\"},{\"content\":{\"connectorIds\":[\"RConn1\",\"RConn2\",\"RConn3\",\"RConn4\"],\"side\":\"RIGHT\"},\"type\":\"ConnectorPlacement.EquallySpacedRectSide\",\"uuid\":\"3f5067af-896c-4e1f-b6f7-733e5cdc76c1\"},{\"content\":{\"connectorIds\":[\"In1\",\"In2\"],\"side\":\"TOP\"},\"type\":\"ConnectorPlacement.EquallySpacedRectSide\",\"uuid\":\"f222cd72-c1be-4f44-b61b-d0eaed55e8e5\"},{\"content\":{\"connectorIds\":[],\"side\":\"BOTTOM\"},\"type\":\"ConnectorPlacement.EquallySpacedRectSide\",\"uuid\":\"38c9aab2-4887-46b3-83a5-02a238a37665\"}]},\"type\":\"ConnectorPlacement.EquallySpacedConnector\",\"uuid\":\"8be83150-dffc-4bc0-b134-d817f89340a9\"}],\"packageUris\":[\"http://schema.mathworks.com/mf0/Connector/R2020b\"],\"version\":\"1.0\"}"
  +1 : PMIOPort  Side=Right
  -1 : PMIOPort  Port=2  Side=Right
  +2 : PMIOPort  Port=3  Side=Right
  -2 : PMIOPort  Port=4  Side=Right
  tag scope: P2P_A=global, P2P_B=global
  wires:
  Current Measurement/1 -> [P2P_A]
  P2PSwitchAtoB/1 -> P2P Switch/1(P2PSwitchAtoB)
  Current Measurement1/1 -> [P2P_B]
  P2PSwitchBtoA/1 -> P2P Switch/2(P2PSwitchBtoA)
  connections:
  P2P Switch/RConn1 -- Current Measurement/LConn1
  Current Measurement/RConn1 -- +1/RConn1
  P2P Switch/RConn2 -- -1/RConn1
  Current Measurement1/LConn1 -- P2P Switch/RConn3
  P2P Switch/RConn4 -- -2/RConn1
  Current Measurement1/RConn1 -- +2/RConn1
